simulink model "LaptopTest"  (R2015b)
settings: Solver=VariableStepAuto  StartTime=0.0  StopTime=inf  RelTol=1e-3
libraries: aerolibanimutils x1, simulink x1, dspnetwork x1
(part 2 of 4)

== matlab function LaptopTest/Sensor Generator /MATLAB Function8 ==
  data: value input; output output uint8 size=18; identifier parameter double
function output = data_serialize(value, identifier)

id_ser = sensor_serialize(identifier);
value_ser = sensor_serialize(value);

output = [
    id_ser;
    value_ser;
    ];
end


function m = sensor_serialize(v)
    % dispatch according to type
    if isnumeric(v) 
        m = serialize_numeric(v);
    elseif ischar(v)
        m = serialize_string(v);
    elseif islogical(v)
        m = serialize_logical(v);
	else
		error('Unsupported data type');
    end
end

% single scalar
function m = serialize_scalar(v)
    % Data type & data
    m = [class2tag(class(v)); typecast(v,'uint8').'];
end

% char arrays
function m = serialize_string(v)
    if size(v,1) == 1
        % horizontal string: Type, Length, and Data
        m = [uint8(0); typecast(uint32(length(v)),'uint8').'; uint8(v(:))];
    elseif sum(size(v)) == 0
        % '': special encoding
        m = uint8(200);
    else
        % general char array: Tag & Number of dimensions, Dimensions, Data
        m = [uint8(132); ndims(v); typecast(uint32(size(v)),'uint8').'; uint8(v(:))];
    end
end

% logical arrays
function m = serialize_logical(v)
    % Tag & Number of dimensions, Dimensions, Data
    m = [uint8(133); ndims(v); typecast(uint32(size(v)),'uint8').'; uint8(v(:))];
end

% non-complex and non-sparse numerical matrix
function m = serialize_numeric_simple(v)
    % Tag & Number of dimensions, Dimensions, Data
    m = [16+class2tag(class(v)); ndims(v); typecast(uint32(size(v)),'uint8').'; typecast(v(:).','uint8').'];
end

% Numeric Matrix: can be real/complex, sparse/full, scalar
function m = serialize_numeric(v)
    if issparse(v)
        % Data Type & Dimensions
        m = [uint8(130); typecast(uint64(size(v,1)), 'uint8').'; typecast(uint64(size(v,2)), 'uint8').']; % vectorize
        % Index vectors
        [i,j,s] = find(v);        
        % Real/Complex
        if isreal(v)
            m = [m; serialize_numeric_simple(i); serialize_numeric_simple(j); 1; serialize_numeric_simple(s)];
        else
            m = [m; serialize_numeric_simple(i); serialize_numeric_simple(j); 0; serialize_numeric_simple(real(s)); serialize_numeric_simple(imag(s))];
        end
    elseif ~isreal(v)
        % Data type & contents
        m = [uint8(131); serialize_numeric_simple(real(v)); serialize_numeric_simple(imag(v))];
    elseif isscalar(v)
        % Scalar
        m = serialize_scalar(v);
    else
        % Simple matrix
        m = serialize_numeric_simple(v);
    end
end

% *container* class to byte
function b = class2tag(cls)
	switch cls
		case 'string'
            b = uint8(0);
		case 'double'
			b = uint8(1);
		case 'single'
			b = uint8(2);
		case 'int8'
			b = uint8(3);
		case 'uint8'
			b = uint8(4);
		case 'int16'
			b = uint8(5);
		case 'uint16'
			b = uint8(6);
		case 'int32'
			b = uint8(7);
		case 'uint32'
			b = uint8(8);
		case 'int64'
			b = uint8(9);
		case 'uint64'
			b = uint8(10);
		otherwise
			error('Unknown class');
    end
end

== matlab function LaptopTest/Sensor Generator /MATLAB Function9 ==
  data: value input; output output uint8 size=18; identifier parameter double
function output = data_serialize(value, identifier)

id_ser = sensor_serialize(identifier);
value_ser = sensor_serialize(value);

output = [
    id_ser;
    value_ser;
    ];
end


function m = sensor_serialize(v)
    % dispatch according to type
    if isnumeric(v) 
        m = serialize_numeric(v);
    elseif ischar(v)
        m = serialize_string(v);
    elseif islogical(v)
        m = serialize_logical(v);
	else
		error('Unsupported data type');
    end
end

% single scalar
function m = serialize_scalar(v)
    % Data type & data
    m = [class2tag(class(v)); typecast(v,'uint8').'];
end

% char arrays
function m = serialize_string(v)
    if size(v,1) == 1
        % horizontal string: Type, Length, and Data
        m = [uint8(0); typecast(uint32(length(v)),'uint8').'; uint8(v(:))];
    elseif sum(size(v)) == 0
        % '': special encoding
        m = uint8(200);
    else
        % general char array: Tag & Number of dimensions, Dimensions, Data
        m = [uint8(132); ndims(v); typecast(uint32(size(v)),'uint8').'; uint8(v(:))];
    end
end

% logical arrays
function m = serialize_logical(v)
    % Tag & Number of dimensions, Dimensions, Data
    m = [uint8(133); ndims(v); typecast(uint32(size(v)),'uint8').'; uint8(v(:))];
end

% non-complex and non-sparse numerical matrix
function m = serialize_numeric_simple(v)
    % Tag & Number of dimensions, Dimensions, Data
    m = [16+class2tag(class(v)); ndims(v); typecast(uint32(size(v)),'uint8').'; typecast(v(:).','uint8').'];
end

% Numeric Matrix: can be real/complex, sparse/full, scalar
function m = serialize_numeric(v)
    if issparse(v)
        % Data Type & Dimensions
        m = [uint8(130); typecast(uint64(size(v,1)), 'uint8').'; typecast(uint64(size(v,2)), 'uint8').']; % vectorize
        % Index vectors
        [i,j,s] = find(v);        
        % Real/Complex
        if isreal(v)
            m = [m; serialize_numeric_simple(i); serialize_numeric_simple(j); 1; serialize_numeric_simple(s)];
        else
            m = [m; serialize_numeric_simple(i); serialize_numeric_simple(j); 0; serialize_numeric_simple(real(s)); serialize_numeric_simple(imag(s))];
        end
    elseif ~isreal(v)
        % Data type & contents
        m = [uint8(131); serialize_numeric_simple(real(v)); serialize_numeric_simple(imag(v))];
    elseif isscalar(v)
        % Scalar
        m = serialize_scalar(v);
    else
        % Simple matrix
        m = serialize_numeric_simple(v);
    end
end

% *container* class to byte
function b = class2tag(cls)
	switch cls
		case 'string'
            b = uint8(0);
		case 'double'
			b = uint8(1);
		case 'single'
			b = uint8(2);
		case 'int8'
			b = uint8(3);
		case 'uint8'
			b = uint8(4);
		case 'int16'
			b = uint8(5);
		case 'uint16'
			b = uint8(6);
		case 'int32'
			b = uint8(7);
		case 'uint32'
			b = uint8(8);
		case 'int64'
			b = uint8(9);
		case 'uint64'
			b = uint8(10);
		otherwise
			error('Unknown class');
    end
end

== matlab function LaptopTest/Sensor Generator /MATLAB Function10 ==
  data: value input; output output uint8 size=18; identifier parameter double
function output = data_serialize(value, identifier)

id_ser = sensor_serialize(identifier);
value_ser = sensor_serialize(value);

output = [
    id_ser;
    value_ser;
    ];
end


function m = sensor_serialize(v)
    % dispatch according to type
    if isnumeric(v) 
        m = serialize_numeric(v);
    elseif ischar(v)
        m = serialize_string(v);
    elseif islogical(v)
        m = serialize_logical(v);
	else
		error('Unsupported data type');
    end
end

% single scalar
function m = serialize_scalar(v)
    % Data type & data
    m = [class2tag(class(v)); typecast(v,'uint8').'];
end

% char arrays
function m = serialize_string(v)
    if size(v,1) == 1
        % horizontal string: Type, Length, and Data
        m = [uint8(0); typecast(uint32(length(v)),'uint8').'; uint8(v(:))];
    elseif sum(size(v)) == 0
        % '': special encoding
        m = uint8(200);
    else
        % general char array: Tag & Number of dimensions, Dimensions, Data
        m = [uint8(132); ndims(v); typecast(uint32(size(v)),'uint8').'; uint8(v(:))];
    end
end

% logical arrays
function m = serialize_logical(v)
    % Tag & Number of dimensions, Dimensions, Data
    m = [uint8(133); ndims(v); typecast(uint32(size(v)),'uint8').'; uint8(v(:))];
end

% non-complex and non-sparse numerical matrix
function m = serialize_numeric_simple(v)
    % Tag & Number of dimensions, Dimensions, Data
    m = [16+class2tag(class(v)); ndims(v); typecast(uint32(size(v)),'uint8').'; typecast(v(:).','uint8').'];
end

% Numeric Matrix: can be real/complex, sparse/full, scalar
function m = serialize_numeric(v)
    if issparse(v)
        % Data Type & Dimensions
        m = [uint8(130); typecast(uint64(size(v,1)), 'uint8').'; typecast(uint64(size(v,2)), 'uint8').']; % vectorize
        % Index vectors
        [i,j,s] = find(v);        
        % Real/Complex
        if isreal(v)
            m = [m; serialize_numeric_simple(i); serialize_numeric_simple(j); 1; serialize_numeric_simple(s)];
        else
            m = [m; serialize_numeric_simple(i); serialize_numeric_simple(j); 0; serialize_numeric_simple(real(s)); serialize_numeric_simple(imag(s))];
        end
    elseif ~isreal(v)
        % Data type & contents
        m = [uint8(131); serialize_numeric_simple(real(v)); serialize_numeric_simple(imag(v))];
    elseif isscalar(v)
        % Scalar
        m = serialize_scalar(v);
    else
        % Simple matrix
        m = serialize_numeric_simple(v);
    end
end

% *container* class to byte
function b = class2tag(cls)
	switch cls
		case 'string'
            b = uint8(0);
		case 'double'
			b = uint8(1);
		case 'single'
			b = uint8(2);
		case 'int8'
			b = uint8(3);
		case 'uint8'
			b = uint8(4);
		case 'int16'
			b = uint8(5);
		case 'uint16'
			b = uint8(6);
		case 'int32'
			b = uint8(7);
		case 'uint32'
			b = uint8(8);
		case 'int64'
			b = uint8(9);
		case 'uint64'
			b = uint8(10);
		otherwise
			error('Unknown class');
    end
end

== matlab function LaptopTest/Sensor Generator /MATLAB Function11 ==
  data: value input; output output uint8 size=18; identifier parameter double
function output = data_serialize(value, identifier)

id_ser = sensor_serialize(identifier);
value_ser = sensor_serialize(value);

output = [
    id_ser;
    value_ser;
    ];
end


function m = sensor_serialize(v)
    % dispatch according to type
    if isnumeric(v) 
        m = serialize_numeric(v);
    elseif ischar(v)
        m = serialize_string(v);
    elseif islogical(v)
        m = serialize_logical(v);
	else
		error('Unsupported data type');
    end
end

% single scalar
function m = serialize_scalar(v)
    % Data type & data
    m = [class2tag(class(v)); typecast(v,'uint8').'];
end

% char arrays
function m = serialize_string(v)
    if size(v,1) == 1
        % horizontal string: Type, Length, and Data
        m = [uint8(0); typecast(uint32(length(v)),'uint8').'; uint8(v(:))];
    elseif sum(size(v)) == 0
        % '': special encoding
        m = uint8(200);
    else
        % general char array: Tag & Number of dimensions, Dimensions, Data
        m = [uint8(132); ndims(v); typecast(uint32(size(v)),'uint8').'; uint8(v(:))];
    end
end

% logical arrays
function m = serialize_logical(v)
    % Tag & Number of dimensions, Dimensions, Data
    m = [uint8(133); ndims(v); typecast(uint32(size(v)),'uint8').'; uint8(v(:))];
end

% non-complex and non-sparse numerical matrix
function m = serialize_numeric_simple(v)
    % Tag & Number of dimensions, Dimensions, Data
    m = [16+class2tag(class(v)); ndims(v); typecast(uint32(size(v)),'uint8').'; typecast(v(:).','uint8').'];
end

% Numeric Matrix: can be real/complex, sparse/full, scalar
function m = serialize_numeric(v)
    if issparse(v)
        % Data Type & Dimensions
        m = [uint8(130); typecast(uint64(size(v,1)), 'uint8').'; typecast(uint64(size(v,2)), 'uint8').']; % vectorize
        % Index vectors
        [i,j,s] = find(v);        
        % Real/Complex
        if isreal(v)
            m = [m; serialize_numeric_simple(i); serialize_numeric_simple(j); 1; serialize_numeric_simple(s)];
        else
            m = [m; serialize_numeric_simple(i); serialize_numeric_simple(j); 0; serialize_numeric_simple(real(s)); serialize_numeric_simple(imag(s))];
        end
    elseif ~isreal(v)
        % Data type & contents
        m = [uint8(131); serialize_numeric_simple(real(v)); serialize_numeric_simple(imag(v))];
    elseif isscalar(v)
        % Scalar
        m = serialize_scalar(v);
    else
        % Simple matrix
        m = serialize_numeric_simple(v);
    end
end

% *container* class to byte
function b = class2tag(cls)
	switch cls
		case 'string'
            b = uint8(0);
		case 'double'
			b = uint8(1);
		case 'single'
			b = uint8(2);
		case 'int8'
			b = uint8(3);
		case 'uint8'
			b = uint8(4);
		case 'int16'
			b = uint8(5);
		case 'uint16'
			b = uint8(6);
		case 'int32'
			b = uint8(7);
		case 'uint32'
			b = uint8(8);
		case 'int64'
			b = uint8(9);
		case 'uint64'
			b = uint8(10);
		otherwise
			error('Unknown class');
    end
end

== matlab function LaptopTest/Sensor Generator /MATLAB Function12 ==
  data: value input; output output uint8 size=18; identifier parameter double
function output = data_serialize(value, identifier)

id_ser = sensor_serialize(identifier);
value_ser = sensor_serialize(value);

output = [
    id_ser;
    value_ser;
    ];
end


function m = sensor_serialize(v)
    % dispatch according to type
    if isnumeric(v) 
        m = serialize_numeric(v);
    elseif ischar(v)
        m = serialize_string(v);
    elseif islogical(v)
        m = serialize_logical(v);
	else
		error('Unsupported data type');
    end
end

% single scalar
function m = serialize_scalar(v)
    % Data type & data
    m = [class2tag(class(v)); typecast(v,'uint8').'];
end

% char arrays
function m = serialize_string(v)
    if size(v,1) == 1
        % horizontal string: Type, Length, and Data
        m = [uint8(0); typecast(uint32(length(v)),'uint8').'; uint8(v(:))];
    elseif sum(size(v)) == 0
        % '': special encoding
        m = uint8(200);
    else
        % general char array: Tag & Number of dimensions, Dimensions, Data
        m = [uint8(132); ndims(v); typecast(uint32(size(v)),'uint8').'; uint8(v(:))];
    end
end

% logical arrays
function m = serialize_logical(v)
    % Tag & Number of dimensions, Dimensions, Data
    m = [uint8(133); ndims(v); typecast(uint32(size(v)),'uint8').'; uint8(v(:))];
end

% non-complex and non-sparse numerical matrix
function m = serialize_numeric_simple(v)
    % Tag & Number of dimensions, Dimensions, Data
    m = [16+class2tag(class(v)); ndims(v); typecast(uint32(size(v)),'uint8').'; typecast(v(:).','uint8').'];
end

% Numeric Matrix: can be real/complex, sparse/full, scalar
function m = serialize_numeric(v)
    if issparse(v)
        % Data Type & Dimensions
        m = [uint8(130); typecast(uint64(size(v,1)), 'uint8').'; typecast(uint64(size(v,2)), 'uint8').']; % vectorize
        % Index vectors
        [i,j,s] = find(v);        
        % Real/Complex
        if isreal(v)
            m = [m; serialize_numeric_simple(i); serialize_numeric_simple(j); 1; serialize_numeric_simple(s)];
        else
            m = [m; serialize_numeric_simple(i); serialize_numeric_simple(j); 0; serialize_numeric_simple(real(s)); serialize_numeric_simple(imag(s))];
        end
    elseif ~isreal(v)
        % Data type & contents
        m = [uint8(131); serialize_numeric_simple(real(v)); serialize_numeric_simple(imag(v))];
    elseif isscalar(v)
        % Scalar
        m = serialize_scalar(v);
    else
        % Simple matrix
        m = serialize_numeric_simple(v);
    end
end

% *container* class to byte
function b = class2tag(cls)
	switch cls
		case 'string'
            b = uint8(0);
		case 'double'
			b = uint8(1);
		case 'single'
			b = uint8(2);
		case 'int8'
			b = uint8(3);
		case 'uint8'
			b = uint8(4);
		case 'int16'
			b = uint8(5);
		case 'uint16'
			b = uint8(6);
		case 'int32'
			b = uint8(7);
		case 'uint32'
			b = uint8(8);
		case 'int64'
			b = uint8(9);
		case 'uint64'
			b = uint8(10);
		otherwise
			error('Unknown class');
    end
end

== matlab function LaptopTest/Sensor Generator /MATLAB Function13 ==
  data: value input; output output uint8 size=18; identifier parameter double
function output = data_serialize(value, identifier)

id_ser = sensor_serialize(identifier);
value_ser = sensor_serialize(value);

output = [
    id_ser;
    value_ser;
    ];
end


function m = sensor_serialize(v)
    % dispatch according to type
    if isnumeric(v) 
        m = serialize_numeric(v);
    elseif ischar(v)
        m = serialize_string(v);
    elseif islogical(v)
        m = serialize_logical(v);
	else
		error('Unsupported data type');
    end
end

% single scalar
function m = serialize_scalar(v)
    % Data type & data
    m = [class2tag(class(v)); typecast(v,'uint8').'];
end

% char arrays
function m = serialize_string(v)
    if size(v,1) == 1
        % horizontal string: Type, Length, and Data
        m = [uint8(0); typecast(uint32(length(v)),'uint8').'; uint8(v(:))];
    elseif sum(size(v)) == 0
        % '': special encoding
        m = uint8(200);
    else
        % general char array: Tag & Number of dimensions, Dimensions, Data
        m = [uint8(132); ndims(v); typecast(uint32(size(v)),'uint8').'; uint8(v(:))];
    end
end

% logical arrays
function m = serialize_logical(v)
    % Tag & Number of dimensions, Dimensions, Data
    m = [uint8(133); ndims(v); typecast(uint32(size(v)),'uint8').'; uint8(v(:))];
end

% non-complex and non-sparse numerical matrix
function m = serialize_numeric_simple(v)
    % Tag & Number of dimensions, Dimensions, Data
    m = [16+class2tag(class(v)); ndims(v); typecast(uint32(size(v)),'uint8').'; typecast(v(:).','uint8').'];
end

% Numeric Matrix: can be real/complex, sparse/full, scalar
function m = serialize_numeric(v)
    if issparse(v)
        % Data Type & Dimensions
        m = [uint8(130); typecast(uint64(size(v,1)), 'uint8').'; typecast(uint64(size(v,2)), 'uint8').']; % vectorize
        % Index vectors
        [i,j,s] = find(v);        
        % Real/Complex
        if isreal(v)
            m = [m; serialize_numeric_simple(i); serialize_numeric_simple(j); 1; serialize_numeric_simple(s)];
        else
            m = [m; serialize_numeric_simple(i); serialize_numeric_simple(j); 0; serialize_numeric_simple(real(s)); serialize_numeric_simple(imag(s))];
        end
    elseif ~isreal(v)
        % Data type & contents
        m = [uint8(131); serialize_numeric_simple(real(v)); serialize_numeric_simple(imag(v))];
    elseif isscalar(v)
        % Scalar
        m = serialize_scalar(v);
    else
        % Simple matrix
        m = serialize_numeric_simple(v);
    end
end

% *container* class to byte
function b = class2tag(cls)
	switch cls
		case 'string'
            b = uint8(0);
		case 'double'
			b = uint8(1);
		case 'single'
			b = uint8(2);
		case 'int8'
			b = uint8(3);
		case 'uint8'
			b = uint8(4);
		case 'int16'
			b = uint8(5);
		case 'uint16'
			b = uint8(6);
		case 'int32'
			b = uint8(7);
		case 'uint32'
			b = uint8(8);
		case 'int64'
			b = uint8(9);
		case 'uint64'
			b = uint8(10);
		otherwise
			error('Unknown class');
    end
end

== matlab function LaptopTest/Sensor Generator /MATLAB Function14 ==
  data: value input; output output uint8 size=18; identifier parameter double
function output = data_serialize(value, identifier)

id_ser = sensor_serialize(identifier);
value_ser = sensor_serialize(value);

output = [
    id_ser;
    value_ser;
    ];
end


function m = sensor_serialize(v)
    % dispatch according to type
    if isnumeric(v) 
        m = serialize_numeric(v);
    elseif ischar(v)
        m = serialize_string(v);
    elseif islogical(v)
        m = serialize_logical(v);
	else
		error('Unsupported data type');
    end
end

% single scalar
function m = serialize_scalar(v)
    % Data type & data
    m = [class2tag(class(v)); typecast(v,'uint8').'];
end

% char arrays
function m = serialize_string(v)
    if size(v,1) == 1
        % horizontal string: Type, Length, and Data
        m = [uint8(0); typecast(uint32(length(v)),'uint8').'; uint8(v(:))];
    elseif sum(size(v)) == 0
        % '': special encoding
        m = uint8(200);
    else
        % general char array: Tag & Number of dimensions, Dimensions, Data
        m = [uint8(132); ndims(v); typecast(uint32(size(v)),'uint8').'; uint8(v(:))];
    end
end

% logical arrays
function m = serialize_logical(v)
    % Tag & Number of dimensions, Dimensions, Data
    m = [uint8(133); ndims(v); typecast(uint32(size(v)),'uint8').'; uint8(v(:))];
end

% non-complex and non-sparse numerical matrix
function m = serialize_numeric_simple(v)
    % Tag & Number of dimensions, Dimensions, Data
    m = [16+class2tag(class(v)); ndims(v); typecast(uint32(size(v)),'uint8').'; typecast(v(:).','uint8').'];
end

% Numeric Matrix: can be real/complex, sparse/full, scalar
function m = serialize_numeric(v)
    if issparse(v)
        % Data Type & Dimensions
        m = [uint8(130); typecast(uint64(size(v,1)), 'uint8').'; typecast(uint64(size(v,2)), 'uint8').']; % vectorize
        % Index vectors
        [i,j,s] = find(v);        
        % Real/Complex
        if isreal(v)
            m = [m; serialize_numeric_simple(i); serialize_numeric_simple(j); 1; serialize_numeric_simple(s)];
        else
            m = [m; serialize_numeric_simple(i); serialize_numeric_simple(j); 0; serialize_numeric_simple(real(s)); serialize_numeric_simple(imag(s))];
        end
    elseif ~isreal(v)
        % Data type & contents
        m = [uint8(131); serialize_numeric_simple(real(v)); serialize_numeric_simple(imag(v))];
    elseif isscalar(v)
        % Scalar
        m = serialize_scalar(v);
    else
        % Simple matrix
        m = serialize_numeric_simple(v);
    end
end

% *container* class to byte
function b = class2tag(cls)
	switch cls
		case 'string'
            b = uint8(0);
		case 'double'
			b = uint8(1);
		case 'single'
			b = uint8(2);
		case 'int8'
			b = uint8(3);
		case 'uint8'
			b = uint8(4);
		case 'int16'
			b = uint8(5);
		case 'uint16'
			b = uint8(6);
		case 'int32'
			b = uint8(7);
		case 'uint32'
			b = uint8(8);
		case 'int64'
			b = uint8(9);
		case 'uint64'
			b = uint8(10);
		otherwise
			error('Unknown class');
    end
end

== matlab function LaptopTest/Sensor Generator /MATLAB Function15 ==
  data: value input; output output uint8 size=18; identifier parameter double
function output = data_serialize(value, identifier)

id_ser = sensor_serialize(identifier);
value_ser = sensor_serialize(value);

output = [
    id_ser;
    value_ser;
    ];
end


function m = sensor_serialize(v)
    % dispatch according to type
    if isnumeric(v) 
        m = serialize_numeric(v);
    elseif ischar(v)
        m = serialize_string(v);
    elseif islogical(v)
        m = serialize_logical(v);
	else
		error('Unsupported data type');
    end
end

% single scalar
function m = serialize_scalar(v)
    % Data type & data
    m = [class2tag(class(v)); typecast(v,'uint8').'];
end

% char arrays
function m = serialize_string(v)
    if size(v,1) == 1
        % horizontal string: Type, Length, and Data
        m = [uint8(0); typecast(uint32(length(v)),'uint8').'; uint8(v(:))];
    elseif sum(size(v)) == 0
        % '': special encoding
        m = uint8(200);
    else
        % general char array: Tag & Number of dimensions, Dimensions, Data
        m = [uint8(132); ndims(v); typecast(uint32(size(v)),'uint8').'; uint8(v(:))];
    end
end

% logical arrays
function m = serialize_logical(v)
    % Tag & Number of dimensions, Dimensions, Data
    m = [uint8(133); ndims(v); typecast(uint32(size(v)),'uint8').'; uint8(v(:))];
end

% non-complex and non-sparse numerical matrix
function m = serialize_numeric_simple(v)
    % Tag & Number of dimensions, Dimensions, Data
    m = [16+class2tag(class(v)); ndims(v); typecast(uint32(size(v)),'uint8').'; typecast(v(:).','uint8').'];
end

% Numeric Matrix: can be real/complex, sparse/full, scalar
function m = serialize_numeric(v)
    if issparse(v)
        % Data Type & Dimensions
        m = [uint8(130); typecast(uint64(size(v,1)), 'uint8').'; typecast(uint64(size(v,2)), 'uint8').']; % vectorize
        % Index vectors
        [i,j,s] = find(v);        
        % Real/Complex
        if isreal(v)
            m = [m; serialize_numeric_simple(i); serialize_numeric_simple(j); 1; serialize_numeric_simple(s)];
        else
            m = [m; serialize_numeric_simple(i); serialize_numeric_simple(j); 0; serialize_numeric_simple(real(s)); serialize_numeric_simple(imag(s))];
        end
    elseif ~isreal(v)
        % Data type & contents
        m = [uint8(131); serialize_numeric_simple(real(v)); serialize_numeric_simple(imag(v))];
    elseif isscalar(v)
        % Scalar
        m = serialize_scalar(v);
    else
        % Simple matrix
        m = serialize_numeric_simple(v);
    end
end

% *container* class to byte
function b = class2tag(cls)
	switch cls
		case 'string'
            b = uint8(0);
		case 'double'
			b = uint8(1);
		case 'single'
			b = uint8(2);
		case 'int8'
			b = uint8(3);
		case 'uint8'
			b = uint8(4);
		case 'int16'
			b = uint8(5);
		case 'uint16'
			b = uint8(6);
		case 'int32'
			b = uint8(7);
		case 'uint32'
			b = uint8(8);
		case 'int64'
			b = uint8(9);
		case 'uint64'
			b = uint8(10);
		otherwise
			error('Unknown class');
    end
end

== matlab function LaptopTest/Sensor Generator /MATLAB Function16 ==
  data: value input; output output uint8 size=18; identifier parameter double
function output = data_serialize(value, identifier)

id_ser = sensor_serialize(identifier);
value_ser = sensor_serialize(value);

output = [
    id_ser;
    value_ser;
    ];
end


function m = sensor_serialize(v)
    % dispatch according to type
    if isnumeric(v) 
        m = serialize_numeric(v);
    elseif ischar(v)
        m = serialize_string(v);
    elseif islogical(v)
        m = serialize_logical(v);
	else
		error('Unsupported data type');
    end
end

% single scalar
function m = serialize_scalar(v)
    % Data type & data
    m = [class2tag(class(v)); typecast(v,'uint8').'];
end

% char arrays
function m = serialize_string(v)
    if size(v,1) == 1
        % horizontal string: Type, Length, and Data
        m = [uint8(0); typecast(uint32(length(v)),'uint8').'; uint8(v(:))];
    elseif sum(size(v)) == 0
        % '': special encoding
        m = uint8(200);
    else
        % general char array: Tag & Number of dimensions, Dimensions, Data
        m = [uint8(132); ndims(v); typecast(uint32(size(v)),'uint8').'; uint8(v(:))];
    end
end

% logical arrays
function m = serialize_logical(v)
    % Tag & Number of dimensions, Dimensions, Data
    m = [uint8(133); ndims(v); typecast(uint32(size(v)),'uint8').'; uint8(v(:))];
end

% non-complex and non-sparse numerical matrix
function m = serialize_numeric_simple(v)
    % Tag & Number of dimensions, Dimensions, Data
    m = [16+class2tag(class(v)); ndims(v); typecast(uint32(size(v)),'uint8').'; typecast(v(:).','uint8').'];
end

% Numeric Matrix: can be real/complex, sparse/full, scalar
function m = serialize_numeric(v)
    if issparse(v)
        % Data Type & Dimensions
        m = [uint8(130); typecast(uint64(size(v,1)), 'uint8').'; typecast(uint64(size(v,2)), 'uint8').']; % vectorize
        % Index vectors
        [i,j,s] = find(v);        
        % Real/Complex
        if isreal(v)
            m = [m; serialize_numeric_simple(i); serialize_numeric_simple(j); 1; serialize_numeric_simple(s)];
        else
            m = [m; serialize_numeric_simple(i); serialize_numeric_simple(j); 0; serialize_numeric_simple(real(s)); serialize_numeric_simple(imag(s))];
        end
    elseif ~isreal(v)
        % Data type & contents
        m = [uint8(131); serialize_numeric_simple(real(v)); serialize_numeric_simple(imag(v))];
    elseif isscalar(v)
        % Scalar
        m = serialize_scalar(v);
    else
        % Simple matrix
        m = serialize_numeric_simple(v);
    end
end

% *container* class to byte
function b = class2tag(cls)
	switch cls
		case 'string'
            b = uint8(0);
		case 'double'
			b = uint8(1);
		case 'single'
			b = uint8(2);
		case 'int8'
			b = uint8(3);
		case 'uint8'
			b = uint8(4);
		case 'int16'
			b = uint8(5);
		case 'uint16'
			b = uint8(6);
		case 'int32'
			b = uint8(7);
		case 'uint32'
			b = uint8(8);
		case 'int64'
			b = uint8(9);
		case 'uint64'
			b = uint8(10);
		otherwise
			error('Unknown class');
    end
end

== matlab function LaptopTest/Sensor Generator /MATLAB Function17 ==
  data: value input; output output uint8 size=18; identifier parameter double
function output = data_serialize(value, identifier)

id_ser = sensor_serialize(identifier);
value_ser = sensor_serialize(value);

output = [
    id_ser;
    value_ser;
    ];
end


function m = sensor_serialize(v)
    % dispatch according to type
    if isnumeric(v) 
        m = serialize_numeric(v);
    elseif ischar(v)
        m = serialize_string(v);
    elseif islogical(v)
        m = serialize_logical(v);
	else
		error('Unsupported data type');
    end
end

% single scalar
function m = serialize_scalar(v)
    % Data type & data
    m = [class2tag(class(v)); typecast(v,'uint8').'];
end

% char arrays
function m = serialize_string(v)
    if size(v,1) == 1
        % horizontal string: Type, Length, and Data
        m = [uint8(0); typecast(uint32(length(v)),'uint8').'; uint8(v(:))];
    elseif sum(size(v)) == 0
        % '': special encoding
        m = uint8(200);
    else
        % general char array: Tag & Number of dimensions, Dimensions, Data
        m = [uint8(132); ndims(v); typecast(uint32(size(v)),'uint8').'; uint8(v(:))];
    end
end

% logical arrays
function m = serialize_logical(v)
    % Tag & Number of dimensions, Dimensions, Data
    m = [uint8(133); ndims(v); typecast(uint32(size(v)),'uint8').'; uint8(v(:))];
end

% non-complex and non-sparse numerical matrix
function m = serialize_numeric_simple(v)
    % Tag & Number of dimensions, Dimensions, Data
    m = [16+class2tag(class(v)); ndims(v); typecast(uint32(size(v)),'uint8').'; typecast(v(:).','uint8').'];
end

% Numeric Matrix: can be real/complex, sparse/full, scalar
function m = serialize_numeric(v)
    if issparse(v)
        % Data Type & Dimensions
        m = [uint8(130); typecast(uint64(size(v,1)), 'uint8').'; typecast(uint64(size(v,2)), 'uint8').']; % vectorize
        % Index vectors
        [i,j,s] = find(v);        
        % Real/Complex
        if isreal(v)
            m = [m; serialize_numeric_simple(i); serialize_numeric_simple(j); 1; serialize_numeric_simple(s)];
        else
            m = [m; serialize_numeric_simple(i); serialize_numeric_simple(j); 0; serialize_numeric_simple(real(s)); serialize_numeric_simple(imag(s))];
        end
    elseif ~isreal(v)
        % Data type & contents
        m = [uint8(131); serialize_numeric_simple(real(v)); serialize_numeric_simple(imag(v))];
    elseif isscalar(v)
        % Scalar
        m = serialize_scalar(v);
    else
        % Simple matrix
        m = serialize_numeric_simple(v);
    end
end

% *container* class to byte
function b = class2tag(cls)
	switch cls
		case 'string'
            b = uint8(0);
		case 'double'
			b = uint8(1);
		case 'single'
			b = uint8(2);
		case 'int8'
			b = uint8(3);
		case 'uint8'
			b = uint8(4);
		case 'int16'
			b = uint8(5);
		case 'uint16'
			b = uint8(6);
		case 'int32'
			b = uint8(7);
		case 'uint32'
			b = uint8(8);
		case 'int64'
			b = uint8(9);
		case 'uint64'
			b = uint8(10);
		otherwise
			error('Unknown class');
    end
end

== matlab function LaptopTest/UDP Packet/MATLAB Function ==
  data: time input; output output
function output = time_serialize(time)

time_ser = serialize(time);
output = time_ser;
end


function m = serialize(v)
    % dispatch according to type
    if isnumeric(v) 
        m = serialize_numeric(v);
    elseif ischar(v)
        m = serialize_string(v);
    elseif islogical(v)
        m = serialize_logical(v);
	else
		error('Unsupported data type');
    end
end

% single scalar
function m = serialize_scalar(v)
    % Data type & data
    m = [class2tag(class(v)); typecast(v,'uint8').'];
end

% char arrays
function m = serialize_string(v)
    if size(v,1) == 1
        % horizontal string: Type, Length, and Data
        m = [uint8(0); typecast(uint32(length(v)),'uint8').'; uint8(v(:))];
    elseif sum(size(v)) == 0
        % '': special encoding
        m = uint8(200);
    else
        % general char array: Tag & Number of dimensions, Dimensions, Data
        m = [uint8(132); ndims(v); typecast(uint32(size(v)),'uint8').'; uint8(v(:))];
    end
end

% logical arrays
function m = serialize_logical(v)
    % Tag & Number of dimensions, Dimensions, Data
    m = [uint8(133); ndims(v); typecast(uint32(size(v)),'uint8').'; uint8(v(:))];
end

% non-complex and non-sparse numerical matrix
function m = serialize_numeric_simple(v)
    % Tag & Number of dimensions, Dimensions, Data
    m = [16+class2tag(class(v)); ndims(v); typecast(uint32(size(v)),'uint8').'; typecast(v(:).','uint8').'];
end

% Numeric Matrix: can be real/complex, sparse/full, scalar
function m = serialize_numeric(v)
    if issparse(v)
        % Data Type & Dimensions
        m = [uint8(130); typecast(uint64(size(v,1)), 'uint8').'; typecast(uint64(size(v,2)), 'uint8').']; % vectorize
        % Index vectors
        [i,j,s] = find(v);        
        % Real/Complex
        if isreal(v)
            m = [m; serialize_numeric_simple(i); serialize_numeric_simple(j); 1; serialize_numeric_simple(s)];
        else
            m = [m; serialize_numeric_simple(i); serialize_numeric_simple(j); 0; serialize_numeric_simple(real(s)); serialize_numeric_simple(imag(s))];
        end
    elseif ~isreal(v)
        % Data type & contents
        m = [uint8(131); serialize_numeric_simple(real(v)); serialize_numeric_simple(imag(v))];
    elseif isscalar(v)
        % Scalar
        m = serialize_scalar(v);
    else
        % Simple matrix
        m = serialize_numeric_simple(v);
    end
end

% *container* class to byte
function b = class2tag(cls)
	switch cls
		case 'string'
            b = uint8(0);
		case 'double'
			b = uint8(1);
		case 'single'
			b = uint8(2);
		case 'int8'
			b = uint8(3);
		case 'uint8'
			b = uint8(4);
		case 'int16'
			b = uint8(5);
		case 'uint16'
			b = uint8(6);
		case 'int32'
			b = uint8(7);
		case 'uint32'
			b = uint8(8);
		case 'int64'
			b = uint8(9);
		case 'uint64'
			b = uint8(10);
		otherwise
			error('Unknown class');
    end
end

== matlab function LaptopTest/Sensor Generator /MATLAB Function18 ==
  data: value input; output output uint8 size=18; identifier parameter double
function output = data_serialize(value, identifier)

id_ser = sensor_serialize(identifier);
value_ser = sensor_serialize(value);

output = [
    id_ser;
    value_ser;
    ];
end


function m = sensor_serialize(v)
    % dispatch according to type
    if isnumeric(v) 
        m = serialize_numeric(v);
    elseif ischar(v)
        m = serialize_string(v);
    elseif islogical(v)
        m = serialize_logical(v);
	else
		error('Unsupported data type');
    end
end

% single scalar
function m = serialize_scalar(v)
    % Data type & data
    m = [class2tag(class(v)); typecast(v,'uint8').'];
end

% char arrays
function m = serialize_string(v)
    if size(v,1) == 1
        % horizontal string: Type, Length, and Data
        m = [uint8(0); typecast(uint32(length(v)),'uint8').'; uint8(v(:))];
    elseif sum(size(v)) == 0
        % '': special encoding
        m = uint8(200);
    else
        % general char array: Tag & Number of dimensions, Dimensions, Data
        m = [uint8(132); ndims(v); typecast(uint32(size(v)),'uint8').'; uint8(v(:))];
    end
end

% logical arrays
function m = serialize_logical(v)
    % Tag & Number of dimensions, Dimensions, Data
    m = [uint8(133); ndims(v); typecast(uint32(size(v)),'uint8').'; uint8(v(:))];
end

% non-complex and non-sparse numerical matrix
function m = serialize_numeric_simple(v)
    % Tag & Number of dimensions, Dimensions, Data
    m = [16+class2tag(class(v)); ndims(v); typecast(uint32(size(v)),'uint8').'; typecast(v(:).','uint8').'];
end

% Numeric Matrix: can be real/complex, sparse/full, scalar
function m = serialize_numeric(v)
    if issparse(v)
        % Data Type & Dimensions
        m = [uint8(130); typecast(uint64(size(v,1)), 'uint8').'; typecast(uint64(size(v,2)), 'uint8').']; % vectorize
        % Index vectors
        [i,j,s] = find(v);        
        % Real/Complex
        if isreal(v)
            m = [m; serialize_numeric_simple(i); serialize_numeric_simple(j); 1; serialize_numeric_simple(s)];
        else
            m = [m; serialize_numeric_simple(i); serialize_numeric_simple(j); 0; serialize_numeric_simple(real(s)); serialize_numeric_simple(imag(s))];
        end
    elseif ~isreal(v)
        % Data type & contents
        m = [uint8(131); serialize_numeric_simple(real(v)); serialize_numeric_simple(imag(v))];
    elseif isscalar(v)
        % Scalar
        m = serialize_scalar(v);
    else
        % Simple matrix
        m = serialize_numeric_simple(v);
    end
end

% *container* class to byte
function b = class2tag(cls)
	switch cls
		case 'string'
            b = uint8(0);
		case 'double'
			b = uint8(1);
		case 'single'
			b = uint8(2);
		case 'int8'
			b = uint8(3);
		case 'uint8'
			b = uint8(4);
		case 'int16'
			b = uint8(5);
		case 'uint16'
			b = uint8(6);
		case 'int32'
			b = uint8(7);
		case 'uint32'
			b = uint8(8);
		case 'int64'
			b = uint8(9);
		case 'uint64'
			b = uint8(10);
		otherwise
			error('Unknown class');
    end
end

== matlab function LaptopTest/Sensor Generator /MATLAB Function19 ==
  data: value input; output output uint8 size=18; identifier parameter double
function output = data_serialize(value, identifier)

id_ser = sensor_serialize(identifier);
value_ser = sensor_serialize(value);

output = [
    id_ser;
    value_ser;
    ];
end


function m = sensor_serialize(v)
    % dispatch according to type
    if isnumeric(v) 
        m = serialize_numeric(v);
    elseif ischar(v)
        m = serialize_string(v);
    elseif islogical(v)
        m = serialize_logical(v);
	else
		error('Unsupported data type');
    end
end

% single scalar
function m = serialize_scalar(v)
    % Data type & data
    m = [class2tag(class(v)); typecast(v,'uint8').'];
end

% char arrays
function m = serialize_string(v)
    if size(v,1) == 1
        % horizontal string: Type, Length, and Data
        m = [uint8(0); typecast(uint32(length(v)),'uint8').'; uint8(v(:))];
    elseif sum(size(v)) == 0
        % '': special encoding
        m = uint8(200);
    else
        % general char array: Tag & Number of dimensions, Dimensions, Data
        m = [uint8(132); ndims(v); typecast(uint32(size(v)),'uint8').'; uint8(v(:))];
    end
end

% logical arrays
function m = serialize_logical(v)
    % Tag & Number of dimensions, Dimensions, Data
    m = [uint8(133); ndims(v); typecast(uint32(size(v)),'uint8').'; uint8(v(:))];
end

% non-complex and non-sparse numerical matrix
function m = serialize_numeric_simple(v)
    % Tag & Number of dimensions, Dimensions, Data
    m = [16+class2tag(class(v)); ndims(v); typecast(uint32(size(v)),'uint8').'; typecast(v(:).','uint8').'];
end

% Numeric Matrix: can be real/complex, sparse/full, scalar
function m = serialize_numeric(v)
    if issparse(v)
        % Data Type & Dimensions
        m = [uint8(130); typecast(uint64(size(v,1)), 'uint8').'; typecast(uint64(size(v,2)), 'uint8').']; % vectorize
        % Index vectors
        [i,j,s] = find(v);        
        % Real/Complex
        if isreal(v)
            m = [m; serialize_numeric_simple(i); serialize_numeric_simple(j); 1; serialize_numeric_simple(s)];
        else
            m = [m; serialize_numeric_simple(i); serialize_numeric_simple(j); 0; serialize_numeric_simple(real(s)); serialize_numeric_simple(imag(s))];
        end
    elseif ~isreal(v)
        % Data type & contents
        m = [uint8(131); serialize_numeric_simple(real(v)); serialize_numeric_simple(imag(v))];
    elseif isscalar(v)
        % Scalar
        m = serialize_scalar(v);
    else
        % Simple matrix
        m = serialize_numeric_simple(v);
    end
end

% *container* class to byte
function b = class2tag(cls)
	switch cls
		case 'string'
            b = uint8(0);
		case 'double'
			b = uint8(1);
		case 'single'
			b = uint8(2);
		case 'int8'
			b = uint8(3);
		case 'uint8'
			b = uint8(4);
		case 'int16'
			b = uint8(5);
		case 'uint16'
			b = uint8(6);
		case 'int32'
			b = uint8(7);
		case 'uint32'
			b = uint8(8);
		case 'int64'
			b = uint8(9);
		case 'uint64'
			b = uint8(10);
		otherwise
			error('Unknown class');
    end
end

== matlab function LaptopTest/Sensor Generator 1/MATLAB Function ==
  data: value input; output output uint8 size=18; identifier parameter double
function output = data_serialize(value, identifier)

id_ser = sensor_serialize(identifier);
value_ser = sensor_serialize(value);

output = [
    id_ser;
    value_ser;
    ];
end


function m = sensor_serialize(v)
    % dispatch according to type
    if isnumeric(v) 
        m = serialize_numeric(v);
    elseif ischar(v)
        m = serialize_string(v);
    elseif islogical(v)
        m = serialize_logical(v);
	else
		error('Unsupported data type');
    end
end

% single scalar
function m = serialize_scalar(v)
    % Data type & data
    m = [class2tag(class(v)); typecast(v,'uint8').'];
end

% char arrays
function m = serialize_string(v)
    if size(v,1) == 1
        % horizontal string: Type, Length, and Data
        m = [uint8(0); typecast(uint32(length(v)),'uint8').'; uint8(v(:))];
    elseif sum(size(v)) == 0
        % '': special encoding
        m = uint8(200);
    else
        % general char array: Tag & Number of dimensions, Dimensions, Data
        m = [uint8(132); ndims(v); typecast(uint32(size(v)),'uint8').'; uint8(v(:))];
    end
end

% logical arrays
function m = serialize_logical(v)
    % Tag & Number of dimensions, Dimensions, Data
    m = [uint8(133); ndims(v); typecast(uint32(size(v)),'uint8').'; uint8(v(:))];
end

% non-complex and non-sparse numerical matrix
function m = serialize_numeric_simple(v)
    % Tag & Number of dimensions, Dimensions, Data
    m = [16+class2tag(class(v)); ndims(v); typecast(uint32(size(v)),'uint8').'; typecast(v(:).','uint8').'];
end

% Numeric Matrix: can be real/complex, sparse/full, scalar
function m = serialize_numeric(v)
    if issparse(v)
        % Data Type & Dimensions
        m = [uint8(130); typecast(uint64(size(v,1)), 'uint8').'; typecast(uint64(size(v,2)), 'uint8').']; % vectorize
        % Index vectors
        [i,j,s] = find(v);        
        % Real/Complex
        if isreal(v)
            m = [m; serialize_numeric_simple(i); serialize_numeric_simple(j); 1; serialize_numeric_simple(s)];
        else
            m = [m; serialize_numeric_simple(i); serialize_numeric_simple(j); 0; serialize_numeric_simple(real(s)); serialize_numeric_simple(imag(s))];
        end
    elseif ~isreal(v)
        % Data type & contents
        m = [uint8(131); serialize_numeric_simple(real(v)); serialize_numeric_simple(imag(v))];
    elseif isscalar(v)
        % Scalar
        m = serialize_scalar(v);
    else
        % Simple matrix
        m = serialize_numeric_simple(v);
    end
end

% *container* class to byte
function b = class2tag(cls)
	switch cls
		case 'string'
            b = uint8(0);
		case 'double'
			b = uint8(1);
		case 'single'
			b = uint8(2);
		case 'int8'
			b = uint8(3);
		case 'uint8'
			b = uint8(4);
		case 'int16'
			b = uint8(5);
		case 'uint16'
			b = uint8(6);
		case 'int32'
			b = uint8(7);
		case 'uint32'
			b = uint8(8);
		case 'int64'
			b = uint8(9);
		case 'uint64'
			b = uint8(10);
		otherwise
			error('Unknown class');
    end
end

== matlab function LaptopTest/Sensor Generator 1/MATLAB Function1 ==
  data: value input; output output uint8 size=18; identifier parameter double
function output = data_serialize(value, identifier)

id_ser = sensor_serialize(identifier);
value_ser = sensor_serialize(value);

output = [
    id_ser;
    value_ser;
    ];
end


function m = sensor_serialize(v)
    % dispatch according to type
    if isnumeric(v) 
        m = serialize_numeric(v);
    elseif ischar(v)
        m = serialize_string(v);
    elseif islogical(v)
        m = serialize_logical(v);
	else
		error('Unsupported data type');
    end
end

% single scalar
function m = serialize_scalar(v)
    % Data type & data
    m = [class2tag(class(v)); typecast(v,'uint8').'];
end

% char arrays
function m = serialize_string(v)
    if size(v,1) == 1
        % horizontal string: Type, Length, and Data
        m = [uint8(0); typecast(uint32(length(v)),'uint8').'; uint8(v(:))];
    elseif sum(size(v)) == 0
        % '': special encoding
        m = uint8(200);
    else
        % general char array: Tag & Number of dimensions, Dimensions, Data
        m = [uint8(132); ndims(v); typecast(uint32(size(v)),'uint8').'; uint8(v(:))];
    end
end

% logical arrays
function m = serialize_logical(v)
    % Tag & Number of dimensions, Dimensions, Data
    m = [uint8(133); ndims(v); typecast(uint32(size(v)),'uint8').'; uint8(v(:))];
end

% non-complex and non-sparse numerical matrix
function m = serialize_numeric_simple(v)
    % Tag & Number of dimensions, Dimensions, Data
    m = [16+class2tag(class(v)); ndims(v); typecast(uint32(size(v)),'uint8').'; typecast(v(:).','uint8').'];
end

% Numeric Matrix: can be real/complex, sparse/full, scalar
function m = serialize_numeric(v)
    if issparse(v)
        % Data Type & Dimensions
        m = [uint8(130); typecast(uint64(size(v,1)), 'uint8').'; typecast(uint64(size(v,2)), 'uint8').']; % vectorize
        % Index vectors
        [i,j,s] = find(v);        
        % Real/Complex
        if isreal(v)
            m = [m; serialize_numeric_simple(i); serialize_numeric_simple(j); 1; serialize_numeric_simple(s)];
        else
            m = [m; serialize_numeric_simple(i); serialize_numeric_simple(j); 0; serialize_numeric_simple(real(s)); serialize_numeric_simple(imag(s))];
        end
    elseif ~isreal(v)
        % Data type & contents
        m = [uint8(131); serialize_numeric_simple(real(v)); serialize_numeric_simple(imag(v))];
    elseif isscalar(v)
        % Scalar
        m = serialize_scalar(v);
    else
        % Simple matrix
        m = serialize_numeric_simple(v);
    end
end

% *container* class to byte
function b = class2tag(cls)
	switch cls
		case 'string'
            b = uint8(0);
		case 'double'
			b = uint8(1);
		case 'single'
			b = uint8(2);
		case 'int8'
			b = uint8(3);
		case 'uint8'
			b = uint8(4);
		case 'int16'
			b = uint8(5);
		case 'uint16'
			b = uint8(6);
		case 'int32'
			b = uint8(7);
		case 'uint32'
			b = uint8(8);
		case 'int64'
			b = uint8(9);
		case 'uint64'
			b = uint8(10);
		otherwise
			error('Unknown class');
    end
end

== matlab function LaptopTest/Sensor Generator 1/MATLAB Function10 ==
  data: value input; output output uint8 size=18; identifier parameter double
function output = data_serialize(value, identifier)

id_ser = sensor_serialize(identifier);
value_ser = sensor_serialize(value);

output = [
    id_ser;
    value_ser;
    ];
end


function m = sensor_serialize(v)
    % dispatch according to type
    if isnumeric(v) 
        m = serialize_numeric(v);
    elseif ischar(v)
        m = serialize_string(v);
    elseif islogical(v)
        m = serialize_logical(v);
	else
		error('Unsupported data type');
    end
end

% single scalar
function m = serialize_scalar(v)
    % Data type & data
    m = [class2tag(class(v)); typecast(v,'uint8').'];
end

% char arrays
function m = serialize_string(v)
    if size(v,1) == 1
        % horizontal string: Type, Length, and Data
        m = [uint8(0); typecast(uint32(length(v)),'uint8').'; uint8(v(:))];
    elseif sum(size(v)) == 0
        % '': special encoding
        m = uint8(200);
    else
        % general char array: Tag & Number of dimensions, Dimensions, Data
        m = [uint8(132); ndims(v); typecast(uint32(size(v)),'uint8').'; uint8(v(:))];
    end
end

% logical arrays
function m = serialize_logical(v)
    % Tag & Number of dimensions, Dimensions, Data
    m = [uint8(133); ndims(v); typecast(uint32(size(v)),'uint8').'; uint8(v(:))];
end

% non-complex and non-sparse numerical matrix
function m = serialize_numeric_simple(v)
    % Tag & Number of dimensions, Dimensions, Data
    m = [16+class2tag(class(v)); ndims(v); typecast(uint32(size(v)),'uint8').'; typecast(v(:).','uint8').'];
end

% Numeric Matrix: can be real/complex, sparse/full, scalar
function m = serialize_numeric(v)
    if issparse(v)
        % Data Type & Dimensions
        m = [uint8(130); typecast(uint64(size(v,1)), 'uint8').'; typecast(uint64(size(v,2)), 'uint8').']; % vectorize
        % Index vectors
        [i,j,s] = find(v);        
        % Real/Complex
        if isreal(v)
            m = [m; serialize_numeric_simple(i); serialize_numeric_simple(j); 1; serialize_numeric_simple(s)];
        else
            m = [m; serialize_numeric_simple(i); serialize_numeric_simple(j); 0; serialize_numeric_simple(real(s)); serialize_numeric_simple(imag(s))];
        end
    elseif ~isreal(v)
        % Data type & contents
        m = [uint8(131); serialize_numeric_simple(real(v)); serialize_numeric_simple(imag(v))];
    elseif isscalar(v)
        % Scalar
        m = serialize_scalar(v);
    else
        % Simple matrix
        m = serialize_numeric_simple(v);
    end
end

% *container* class to byte
function b = class2tag(cls)
	switch cls
		case 'string'
            b = uint8(0);
		case 'double'
			b = uint8(1);
		case 'single'
			b = uint8(2);
		case 'int8'
			b = uint8(3);
		case 'uint8'
			b = uint8(4);
		case 'int16'
			b = uint8(5);
		case 'uint16'
			b = uint8(6);
		case 'int32'
			b = uint8(7);
		case 'uint32'
			b = uint8(8);
		case 'int64'
			b = uint8(9);
		case 'uint64'
			b = uint8(10);
		otherwise
			error('Unknown class');
    end
end
